simulink model "pruebaStateSpaceModel"  (R2022b)
settings: Solver=VariableStepAuto  StartTime=0.0  StopTime=10.0  RelTol=1e-3
values from neighbouring files (symbols this model uses):
  A6 = [0 0 0 0 0 0 0 0 0 0 0 0 ... (100 elements, 10x10)]    [matrices_linealizacion_6gdl.mat]
  B6 = [0 0 0 0 0 0.000575563603666 -0.0459993641186 -0.0505103975277 0.151580453785 0.00175830093621 0 0 ... (80 elements, 10x8)]    [matrices_linealizacion_6gdl.mat]
  C6 = [1 0 0 0 0 0 0 0 0 0 0 1 ... (100 elements, 10x10)]    [matrices_linealizacion_6gdl.mat]
  D6 = [0 0 0 0 0 0 0 0 0 0 0 0 ... (80 elements, 10x8)]    [matrices_linealizacion_6gdl.mat]
settings Model: Creator=ramuj  LastModifiedBy=ramuj

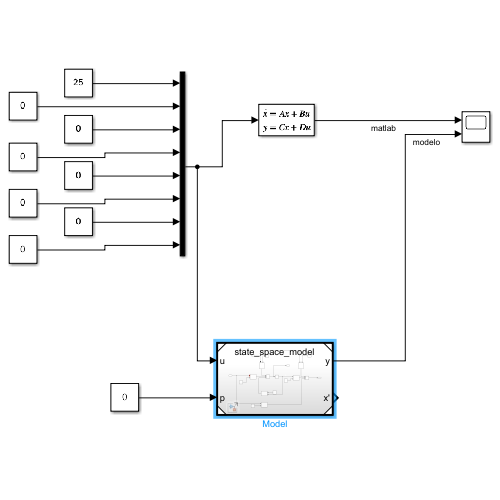
[thumbnail: Simulink's stored preview of the top-level diagram]
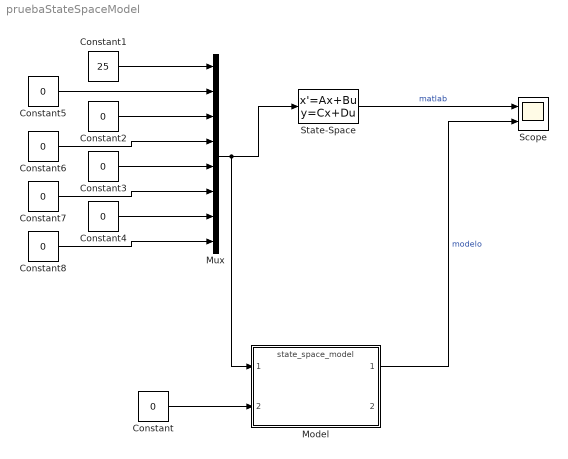
== system pruebaStateSpaceModel ==
  Constant : Constant  Value=0  VectorParams1D=off
  Constant1 : Constant  Value=25
  Constant{2..8} (7 alike) : Constant  Value=0
  Model : ModelReference  ModelNameDialog=state_space_model.slx  SimulationMode=Normal  ModelReferenceVersion=1.7
  Mux : Mux  Inputs=8
  Scope : Scope  NumInputPorts=2
  State-Space : StateSpace  A=A6  B=B6  C=C6  D=D6  InitialCondition=0
  wires:
  Constant/1 -> Model/2
  State-Space/1 -> Scope/1  "matlab"
  Model/1 -> Scope/2  "modelo"
  Constant1/1 -> Mux/1
  Mux/1 -> Model/1, State-Space/1
  Constant5/1 -> Mux/2
  Constant2/1 -> Mux/3
  Constant6/1 -> Mux/4
  Constant3/1 -> Mux/5
  Constant7/1 -> Mux/6
  Constant4/1 -> Mux/7
  Constant8/1 -> Mux/8
